simulink model "fixpt_sl_sum_add"  (Simulink 7.9)
settings: Solver=FixedStepDiscrete  StartTime=0.0  StopTime=0  FixedStep=1  RelTol=1e-3
settings Model: Creator=y_yama  LastModifiedBy=amatsumo
settings DataIOCC: SaveOutput=off  SignalLogging=off  SaveTime=off
settings OptimizationCC: InlineParams=on  InlineInvariantSignals=on  ZeroExternalMemoryAtStartup=off  ZeroInternalMemoryAtStartup=off  InitFltsAndDblsToZero=on  NoFixptDivByZeroProtection=on  EfficientFloat2IntCast=on  OptimizeModelRefInitCode=on  LifeSpan=1
settings DebuggingCC: InheritedTsInSrcMsg=none  FcnCallInpInsideContextMsg=Use local settings  StrictBusMsg=Warning
settings HardwareCC: ProdHWDeviceType=ASIC/FPGA->ASIC/FPGA  TargetEndianess=LittleEndian  TargetHWDeviceType=MATLAB Host  ProdEqTarget=off
settings RTWCC: SystemTargetFile=ert.tlc  GenCodeOnly=on  TemplateMakefile=ert_default_tmf  Description=Real-Time Workshop Embedded Coder (no auto configuration)  GenerateReport=on  ProcessScript=ert_make_rtw_hook  IncludeHyperlinkInReport=on  LaunchReport=on
settings CodeAppCC: GenerateComments=off  IgnoreCustomStorageClasses=off  CustomSymbolStrGlobalVar=$N$M  SimulinkBlockComments=off
settings ERTTargetCC: CodeReplacementLibrary=ANSI_C  MultiwordLength=2048  GenerateSampleERTMain=on  IncludeMdlTerminateFcn=off  SuppressErrorStatus=on  SupportAbsoluteTime=off  SupportNonFinite=off  SupportComplex=off  PurelyIntegerCode=on  InlinedParameterPlacement=NonHierarchical  ERTCustomFileTemplate=example_file_process.tlc  ConvertIfToSwitch=off  SuppressUnreachableDefaultCases=off

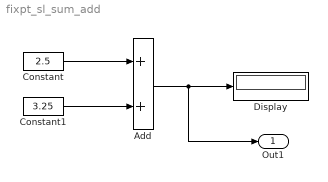
== system fixpt_sl_sum_add ==
  Add : Sum
  Constant : Constant  Value=2.5  OutDataTypeStr=fixdt(1,8,1)  SampleTime=-1
      settings: AttributesFormatString=DataType = %<OutDataTypeStr>
  Constant1 : Constant  Value=3.25  OutDataTypeStr=fixdt(1,8,2)  SampleTime=-1
      settings: AttributesFormatString=DataType = %<OutDataTypeStr>
  Display : Display
      settings: AttributesFormatString=Format = %<Format>
  Out1 : Outport
  wires:
  Add/1 -> Display/1, Out1/1
  Constant/1 -> Add/1
  Constant1/1 -> Add/2
